simulink model "F16ASYM_Controlled_AoA"  (R2012b)
settings: Solver=ode3  SolverMode=SingleTasking  StartTime=0.0  StopTime=inf  FixedStep=T_sim  RelTol=1e-3
InitFcn:
  | load('NN_c_weights_Last_stable.mat')
values from neighbouring files (symbols this model uses):
  K_b_AoA = params(3)    [Cost_function.m]
  K_b_q = params(4)    [Cost_function.m]
  learning = 20    [Scheduling_desing.m]
  Model_used_flag = 1    [Scheduling_desing.m]
  reg_param = 0.5    [Scheduling_desing.m]
  T_sim = 0.02    [Scheduling_desing.m]
  tau_AoA = params(1)    [Cost_function.m]
  tau_q = params(2)    [Cost_function.m]
  Theta_1_roll_last = [0.00183613313267 0.00115998993235 0.0006676025148 0.00194921904952 0.00134963559861 0.00034352059664 0.000447169388141 0.00146749660935 0.00110199952389 7.77922383894e-05 0.00109492833348 0.00192687590535 ... (360 elements, 30x12)]    [NN_i_weights_LAST_STABLE.mat]
  Theta_2_roll_last = [0.000469743069697 0.000355923851088 0.00180035760697 0.00191855117771 0.00118851504447 0.0013331642065 0.0013164316578 0.000643981263341 0.00176817665434 0.000113802099363 0.000426534542462 0.00113815782354 ... (620 elements, 20x31)]    [NN_i_weights_LAST_STABLE.mat]
  Theta_3_roll_last = [9.62071520568e-05 -0.000389870886846 2.08260845013e-05 0.000140787743673 -0.000917525755397 -0.0014324207578 -0.00154701573815 -0.00131544476264 -0.00101205584381 5.06515794689e-05 -0.00111443483676 -0.00143957416141 ... (21 elements, 1x21)]    [NN_i_weights_LAST_STABLE.mat]
  V_long_lastA_w_z = [0.352826086601 -0.253633004548 -0.642535042878 0.237749930435 -0.618390629538 0.858074761295 0.268211230628 -0.448715080196 -0.0406384631192 0.401147605577 0.60598427709 0.0500551915851 ... (300 elements, 30x10)]    [NN_i_weights_LAST_STABLE.mat]
  V_long_lastAoA = [0.0774300162379 0.0911421319631 0.0352371192557 0.0542170286952 0.0651171200844 0.0177112012707 0.0982957728448 0.000259994642558 0.0194724569123 0.0466321328252 0.0556687953852 0.0252668067142 ... (300 elements, 30x10)]    [NN_i_weights_LAST_STABLE.mat]
  V_roll_last = [0.0540918675943 0.0557493347212 0.0839792276608 0.0460576391794 0.0671229058124 0.100220403067 0.0722493281881 0.0648875457457 0.00447599349201 0.0607299103823 0.0488037966361 0.0176785979393 ... (360 elements, 30x12)]    [NN_i_weights_LAST_STABLE.mat]
  V_yaw_last = [0.0965149149679 0.00833616709545 0.0365734360076 0.0523944217566 0.00790252078455 0.0700053845887 0.0345164868709 0.0111568465295 0.094060639546 0.0205483560006 0.000798047494256 0.0862769385758 ... (360 elements, 30x12)]    [NN_i_weights_LAST_STABLE.mat]
  velocity = M_eval_sche(I,J)*a    [Scheduling_desing.m]
  W_long_lastA_w_z = [-0.0522913429974 0.00385484301394 -0.00465489482472 -0.0139416219936 0.00295196421483 -0.013027768541 0.00585545058915 0.00278802233571 -0.00906272782329 -0.000396112031465 0.00405849743321 0.00509668457818 ... (31 elements, 1x31)]    [NN_i_weights_LAST_STABLE.mat]
  W_long_lastAoA = [-0.0192589013922 0.00873109909713 0.00432649597332 0.0420946902441 0.0293366820194 0.0351497798191 0.0234952374236 0.0360841187718 0.0112233388211 0.030147202199 0.0369533138617 0.00218839076415 ... (31 elements, 1x31)]    [NN_i_weights_LAST_STABLE.mat]
  W_roll_last = [-0.0006515532842 0.000535485585715 0.000550946920743 0.000806030945453 0.00045976209382 0.00065557954304 0.000945902185602 0.00070191398535 0.000635215543728 4.66501377412e-05 0.000597079583757 0.000485790566765 ... (31 elements, 1x31)]    [NN_i_weights_LAST_STABLE.mat]
  W_yaw_last = [-4.34263633305e-05 8.83823048922e-05 1.65575463724e-05 3.60293102233e-05 5.19752447623e-05 7.06399280852e-06 7.02425975821e-05 3.62680255076e-05 1.29996379937e-05 8.05072914397e-05 2.39941870661e-05 2.52427840574e-06 ... (31 elements, 1x31)]    [NN_i_weights_LAST_STABLE.mat]
undefined symbols (not defined in the file or in its folder): a1, alpha_map_eval, B, beta_map_eval, C_L_0, DiscIntNeverNeededParam, fi_flag_Simulink, G_eval, H_sq, H_sq_autotrim, k_B, m_B, M_sq, M_sq_autotrim, sigbuilder_block, Stall_curve, trim_control, trim_state, trim_throttle, V_Comp_A_w_z_last, V_Comp_last, V_roll_lastMOD, W_Comp_A_w_z_last, W_Comp_last, W_roll_lastMOD
libraries: Adaptive_FaultTolerantControl x43, dspsigops x29, F16_Actuator_Library x14, simulink x8, aerolibatmos2 x7, dsparch4 x6, simulink_extras x5, aerolibtransform2 x5, qcatlib x4, dspmtrx3 x3, dspvision x2, dspsnks4 x2
(part 5 of 11)

== system F16ASYM_Controlled_AoA/F-16 Non-linear Plant/SYM and ASYM model: No reconfigurable/Actuators Dynamcis ==
  note: Controls:
      | 1. Throttle
      | 2. Elevator_L in deg
      | 3. Elevator_R in deg
      | 4. Aileron_L
      | 5. Aileron_R
      | 6. Rudder
      | 7. LEF_L
      | 8. LEF_R
  note: Units: deg.
  note: Units: deg.
  note: Units: deg.
  note: This addition in LEFs can be done
      |  if assumed Linear aerodynamics
  note: No dynamics for throttle since the engine dynamics is inside the model
  Control_commands : Inport
  Aileron Actuator : F16_Actuator_Library/Aileron Actuator
  Aileron Actuator1 : F16_Actuator_Library/Aileron Actuator
  Aileron_L Trim Setting : Constant  Value=trim_control(2)
  Aileron_R Trim Setting : Constant  Value=-trim_control(2)
  Control Surface Deflections : ToWorkspace  VariableName=surfaces  SampleTime=-1
      settings: Decimation=100
  Demux : Demux  Outputs=8
  Elevator Actuator : F16_Actuator_Library/Elevator Actuator
  Elevator Actuator1 : F16_Actuator_Library/Elevator Actuator
  LEF Actuator : F16_Actuator_Library/LEF Actuator
  LEF Actuator1 : F16_Actuator_Library/LEF Actuator
  Mux{,1,3..7} (7 alike) : Mux  Inputs=2
  Mux2 : Mux  Inputs=8
  Mux8 : Mux  Inputs=7
  Rudder Actuator : F16_Actuator_Library/Rudder Actuator
  Saturation1 : Saturate  UpperLimit=1  LowerLimit=0
  Control Defl Plot : Outport
  Dec_Control_def : Outport  Port=2
  Throttle_meas : Outport  Port=3
  wires:
  Saturation1/1 -> Mux2/1, Throttle_meas/1  "Throttle"
  Aileron_R Trim Setting/1 -> Aileron Actuator1/2
  Aileron_L Trim Setting/1 -> Aileron Actuator/2
  Demux/1 -> Saturation1/1
  Mux7/1 -> [LEF_R]
  LEF Actuator1/1 -> Mux7/2, Mux2/8  "LEF_R"
  Demux/8 -> Mux7/1, LEF Actuator1/1
  Mux6/1 -> [LEF_L]
  LEF Actuator/1 -> Mux2/7, Mux6/2  "LEF_L"
  Demux/7 -> Mux6/1, LEF Actuator/1
  Mux5/1 -> [Ail_R]
  Aileron Actuator1/1 -> Mux2/5, Mux5/1  "Aileron_R"
  Demux/5 -> Aileron Actuator1/1, Mux5/2
  Elevator Actuator1/1 -> Mux2/3, Mux4/1  "Elevator_R"
  Demux/3 -> Mux4/2, Elevator Actuator1/1
  Mux3/1 -> [Rudder]
  Mux1/1 -> [Ail_L]
  Rudder Actuator/1 -> Mux2/6, Mux3/2  "Rudder"
  Aileron Actuator/1 -> Mux2/4, Mux1/2  "Aileron_L"
  Demux/6 -> Mux3/1, Rudder Actuator/1
  Demux/4 -> Aileron Actuator/1, Mux1/1
  Mux/1 -> [Elev_L]
  Elevator Actuator/1 -> Mux2/2, Mux/2  "Elevator_L"
  Mux2/1 -> Control Surface Deflections/1, Dec_Control_def/1
  Demux/2 -> Elevator Actuator/1, Mux/1
  Control_commands/1 -> Demux/1
  Mux8/1 -> Control Defl Plot/1
  [Elev_L] -> Mux8/1
  [Elev_R] -> Mux8/2
  [Ail_L] -> Mux8/3
  [Ail_R] -> Mux8/4
  [Rudder] -> Mux8/5
  [LEF_L] -> Mux8/6
  [LEF_R] -> Mux8/7
  Mux4/1 -> [Elev_R]

== system F16ASYM_Controlled_AoA/F-16 Non-linear Plant/SYM and ASYM model: No reconfigurable/Leading Edge Flap:Symetric deflection ==
  note: Initialize LF_state with -alpha0 value in degrees!!!!
  note: Same as atmos() in nlplant...c
  note: see NASA Technical Paper 1538, p34
  state : Inport
  Bus Selector1 : BusSelector  OutputSignals=X_e,TAS,alpha;beta
  Creating    qbar / ps : Subsystem
  Demux1 : Demux  Outputs=2
  Gain : Gain  Gain=2  SaturateOnIntegerOverflow=on  OutDataTypeStr=Inherit: Same as input  ParamDataTypeStr=Inherit: Same as input
  Gain1 : Gain  Gain=7.25  SaturateOnIntegerOverflow=on  OutDataTypeStr=Inherit: Same as input  ParamDataTypeStr=Inherit: Same as input
  Gain2 : Gain  Gain=1.38  SaturateOnIntegerOverflow=on  OutDataTypeStr=Inherit: Same as input  ParamDataTypeStr=Inherit: Same as input
  LF_state : Integrator  InitialCondition=-trim_state(8)*180/pi
  Selector : Selector  InputPortWidth=3  IndexOptions=Index vector (dialog)  Indices=3  OutputSizes=1
  Sum : Sum  Inputs=-|+|+  SaturateOnIntegerOverflow=on  InputSameDT=on  OutDataTypeStr=Inherit: Same as first input
  Sum1 : Sum  Inputs=|+-  SaturateOnIntegerOverflow=on  InputSameDT=on  OutDataTypeStr=Inherit: Same as first input
  Sum2 : Sum  Inputs=++|  SaturateOnIntegerOverflow=on  InputSameDT=on  OutDataTypeStr=Inherit: Same as first input
  coeff1 : Constant  Value=1.45
  r2d1 : Gain  Gain=180/pi  SaturateOnIntegerOverflow=on  OutDataTypeStr=Inherit: Same as input  ParamDataTypeStr=Inherit: Same as input
  r2d6 : Gain  Gain=9.05  SaturateOnIntegerOverflow=on  OutDataTypeStr=Inherit: Same as input  ParamDataTypeStr=Inherit: Same as input
  delta_lef (deg) : Outport
  wires:
  Bus Selector1/3 -> Demux1/1  "<alpha;beta>"
  Bus Selector1/1 -> Selector/1  "<X_e>"
  r2d6/1 -> Sum/1
  Creating    qbar / ps/1(qbar / ps) -> r2d6/1
  Bus Selector1/2 -> Creating    qbar / ps/2(V)  "<TAS>"
  r2d1/1 -> Gain/1, Sum1/1  "alpha"
  LF_state/1 -> Sum2/2
  Sum2/1 -> Gain2/1, Sum1/2
  coeff1/1 -> Sum/3
  Demux1/1 -> r2d1/1
  Gain2/1 -> Sum/2
  Gain/1 -> Sum2/1
  Gain1/1 -> LF_state/1
  Sum1/1 -> Gain1/1
  state/1 -> Bus Selector1/1
  Sum/1 -> delta_lef (deg)/1
  Selector/1 -> Creating    qbar / ps/1(alt)

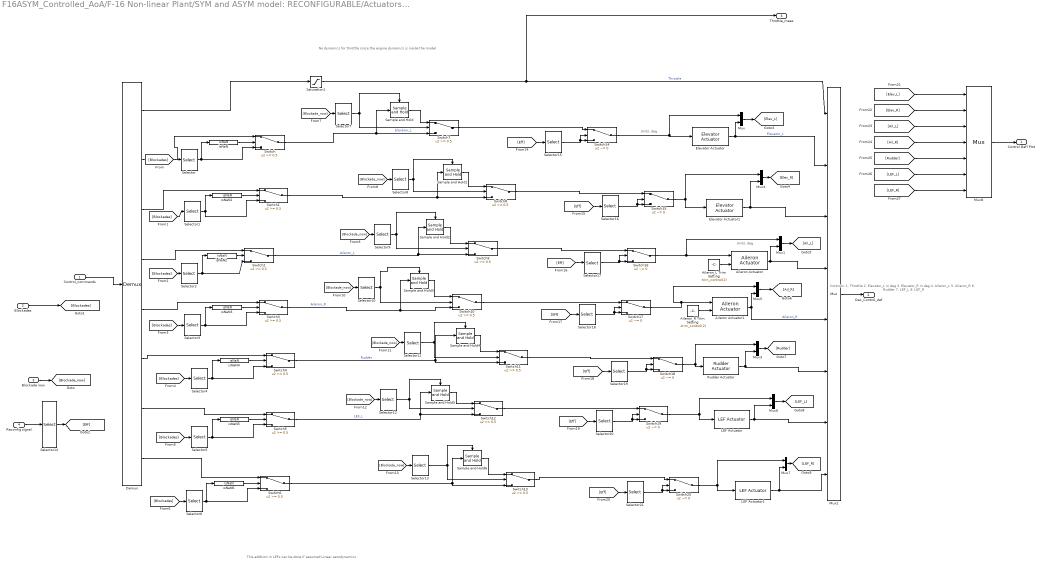
== system F16ASYM_Controlled_AoA/F-16 Non-linear Plant/SYM and ASYM model: RECONFIGURABLE/Actuators Dynamcis ==
  note: No dynamics for throttle since the engine dynamics is inside the model
  note: This addition in LEFs can be done
      |  if assumed Linear aerodynamics
  note: Units: deg.
  note: Units: deg.
  note: Controls:
      | 1. Throttle
      | 2. Elevator_L in deg
      | 3. Elevator_R in deg
      | 4. Aileron_L
      | 5. Aileron_R
      | 6. Rudder
      | 7. LEF_L
      | 8. LEF_R
  Control_commands : Inport
  Blockades : Inport  Port=2
  Blockade now : Inport  Port=3
  Reconfig signal : Inport  Port=4
  Aileron Actuator : F16_Actuator_Library/Aileron Actuator
  Aileron Actuator1 : F16_Actuator_Library/Aileron Actuator
  Aileron_L Trim Setting : Constant  Value=trim_control(2)
  Aileron_R Trim Setting : Constant  Value=-trim_control(2)
  Demux : Demux  Outputs=8
  Elevator Actuator : F16_Actuator_Library/Elevator Actuator
  Elevator Actuator1 : F16_Actuator_Library/Elevator Actuator
  LEF Actuator : F16_Actuator_Library/LEF Actuator
  LEF Actuator1 : F16_Actuator_Library/LEF Actuator
  Mux{,1,3..7} (7 alike) : Mux  Inputs=2
  Mux2 : Mux  Inputs=8
  Mux8 : Mux  Inputs=7
  Rudder Actuator : F16_Actuator_Library/Rudder Actuator
  Sample and Hold : dspsigops/Sample and Hold  trig=Rising edge  initCond=trim_control(1)  latchinput=off
  Sample and Hold1 : dspsigops/Sample and Hold  trig=Rising edge  initCond=trim_control(1)  latchinput=off
  Sample and Hold2 : dspsigops/Sample and Hold  trig=Rising edge  initCond=trim_control(2)  latchinput=off
  Sample and Hold3 : dspsigops/Sample and Hold  trig=Rising edge  initCond=-trim_control(2)  latchinput=off
  Sample and Hold4 : dspsigops/Sample and Hold  trig=Rising edge  initCond=trim_control(3)  latchinput=off
  Sample and Hold5 : dspsigops/Sample and Hold  trig=Rising edge  initCond=dLEF  latchinput=off
  Sample and Hold6 : dspsigops/Sample and Hold  trig=Rising edge  initCond=dLEF  latchinput=off
  Saturation1 : Saturate  UpperLimit=1  LowerLimit=0
  Selector : Selector  InputPortWidth=7  IndexOptions=Index vector (dialog)  Indices=1  OutputSizes=1
  Selector1 : Selector  InputPortWidth=7  IndexOptions=Index vector (dialog)  Indices=2  OutputSizes=1
  Selector10 : Selector  InputPortWidth=7  IndexOptions=Index vector (dialog)  Indices=4  OutputSizes=1
  Selector11 : Selector  InputPortWidth=7  IndexOptions=Index vector (dialog)  Indices=5  OutputSizes=1
  Selector12 : Selector  InputPortWidth=7  IndexOptions=Index vector (dialog)  Indices=6  OutputSizes=1
  Selector13 : Selector  InputPortWidth=7  IndexOptions=Index vector (dialog)  Indices=7  OutputSizes=1
  Selector14 : Selector  InputPortWidth=19  IndexOptions=Index vector (dialog)  Indices=10:16  OutputSizes=1
  Selector15 : Selector  InputPortWidth=7  IndexOptions=Index vector (dialog)  Indices=1  OutputSizes=1
  Selector16 : Selector  InputPortWidth=7  IndexOptions=Index vector (dialog)  Indices=2  OutputSizes=1
  Selector17 : Selector  InputPortWidth=7  IndexOptions=Index vector (dialog)  Indices=3  OutputSizes=1
  Selector18 : Selector  InputPortWidth=7  IndexOptions=Index vector (dialog)  Indices=4  OutputSizes=1
  Selector19 : Selector  InputPortWidth=7  IndexOptions=Index vector (dialog)  Indices=5  OutputSizes=1
  Selector2 : Selector  InputPortWidth=7  IndexOptions=Index vector (dialog)  Indices=3  OutputSizes=1
  Selector20 : Selector  InputPortWidth=7  IndexOptions=Index vector (dialog)  Indices=6  OutputSizes=1
  Selector21 : Selector  InputPortWidth=7  IndexOptions=Index vector (dialog)  Indices=7  OutputSizes=1
  Selector3 : Selector  InputPortWidth=7  IndexOptions=Index vector (dialog)  Indices=4  OutputSizes=1
  Selector4 : Selector  InputPortWidth=7  IndexOptions=Index vector (dialog)  Indices=5  OutputSizes=1
  Selector5 : Selector  InputPortWidth=7  IndexOptions=Index vector (dialog)  Indices=6  OutputSizes=1
  Selector6 : Selector  InputPortWidth=7  IndexOptions=Index vector (dialog)  Indices=7  OutputSizes=1
  Selector7 : Selector  InputPortWidth=7  IndexOptions=Index vector (dialog)  Indices=1  OutputSizes=1
  Selector8 : Selector  InputPortWidth=7  IndexOptions=Index vector (dialog)  Indices=2  OutputSizes=1
  Selector9 : Selector  InputPortWidth=7  IndexOptions=Index vector (dialog)  Indices=3  OutputSizes=1
  Switch{,1..13} (14 alike) : Switch  Threshold=0.5
  Switch{14..20} (7 alike) : Switch  Criteria=u2 ~= 0
  isNaN{,1..6} (7 alike) : RelationalOperator  Operator=isNaN  OutDataTypeStr=boolean
  Control Defl Plot : Outport
  Dec_Control_def : Outport  Port=2
  Throttle_meas : Outport  Port=3
  wires:
  Control_commands/1 -> Demux/1
  Switch14/1 -> Elevator Actuator/1, Mux/1
  Mux2/1 -> Dec_Control_def/1
  Switch16/1 -> Mux1/1, Aileron Actuator/1
  Switch18/1 -> Mux3/1, Rudder Actuator/1
  Switch19/1 -> Mux6/1, LEF Actuator/1
  Switch20/1 -> Mux7/1, LEF Actuator1/1
  Demux/1 -> Saturation1/1
  Aileron_L Trim Setting/1 -> Aileron Actuator/2
  Aileron_R Trim Setting/1 -> Aileron Actuator1/2
  Saturation1/1 -> Mux2/1, Throttle_meas/1  "Throttle"
  Blockades/1 -> [Blockades]
  Blockade now/1 -> [Blockade_now]
  [Blockades] -> Selector/1
  isNaN/1 -> Switch/2
  Demux/2 -> Switch/1
  Selector/1 -> Switch/3, isNaN/1
  [Blockades] -> Selector1/1
  isNaN1/1 -> Switch1/2
  Demux/3 -> Switch1/1
  Selector1/1 -> Switch1/3, isNaN1/1
  [Blockades] -> Selector2/1
  isNaN2/1 -> Switch2/2
  Demux/4 -> Switch2/1
  Selector2/1 -> Switch2/3, isNaN2/1
  [Blockades] -> Selector3/1
  isNaN3/1 -> Switch3/2
  Demux/5 -> Switch3/1
  Selector3/1 -> Switch3/3, isNaN3/1
  [Blockades] -> Selector4/1
  isNaN4/1 -> Switch4/2
  Demux/6 -> Switch4/1
  Selector4/1 -> Switch4/3, isNaN4/1
  [Blockades] -> Selector5/1
  isNaN5/1 -> Switch5/2
  Demux/7 -> Switch5/1
  Selector5/1 -> Switch5/3, isNaN5/1
  [Blockades] -> Selector6/1
  isNaN6/1 -> Switch6/2
  Demux/8 -> Switch6/1
  Selector6/1 -> Switch6/3, isNaN6/1
  Aileron Actuator/1 -> Mux2/4, Mux1/2
  Rudder Actuator/1 -> Mux3/2, Mux2/6
  LEF Actuator/1 -> Mux2/7, Mux6/2
  Switch/1 -> Switch7/3, Sample and Hold/1  "Elevator_L"
  [Blockade_now] -> Selector7/1
  Sample and Hold/1 -> Switch7/1
  Selector7/1 -> Switch7/2, Sample and Hold/Trigger
  Elevator Actuator/1 -> Mux/2, Mux2/2  "Elevator_L"
  Switch1/1 -> Sample and Hold1/1, Switch8/3
  [Blockade_now] -> Selector8/1
  Sample and Hold1/1 -> Switch8/1
  Selector8/1 -> Switch8/2, Sample and Hold1/Trigger
  Switch15/1 -> Mux4/1, Elevator Actuator1/1
  Switch2/1 -> Sample and Hold2/1, Switch9/3  "Aileron_L"
  [Blockade_now] -> Selector9/1
  Sample and Hold2/1 -> Switch9/1
  Selector9/1 -> Sample and Hold2/Trigger, Switch9/2
  Switch17/1 -> Mux5/1, Aileron Actuator1/1
  Aileron Actuator1/1 -> Mux2/5, Mux5/2  "Aileron_R"
  Switch3/1 -> Switch10/3, Sample and Hold3/1  "Aileron_R"
  [Blockade_now] -> Selector10/1
  Sample and Hold3/1 -> Switch10/1
  Selector10/1 -> Sample and Hold3/Trigger, Switch10/2
  Switch4/1 -> Switch11/3, Sample and Hold4/1  "Rudder"
  [Blockade_now] -> Selector11/1
  Sample and Hold4/1 -> Switch11/1
  Selector11/1 -> Switch11/2, Sample and Hold4/Trigger
  Switch5/1 -> Sample and Hold5/1, Switch12/3  "LEF_L"
  [Blockade_now] -> Selector12/1
  Sample and Hold5/1 -> Switch12/1
  Selector12/1 -> Switch12/2, Sample and Hold5/Trigger
  LEF Actuator1/1 -> Mux7/2, Mux2/8
  Switch6/1 -> Switch13/3, Sample and Hold6/1
  [Blockade_now] -> Selector13/1
  Sample and Hold6/1 -> Switch13/1
  Selector13/1 -> Switch13/2, Sample and Hold6/Trigger
  Elevator Actuator1/1 -> Mux4/2, Mux2/3
  Reconfig signal/1 -> Selector14/1
  Selector14/1 -> [Eff]
  [Eff] -> Selector15/1
  Switch7/1 -> Switch14/1
  Selector15/1 -> Switch14/2, Switch14/3
  [Eff] -> Selector16/1
  Switch8/1 -> Switch15/1
  Selector16/1 -> Switch15/2, Switch15/3
  [Eff] -> Selector17/1
  Switch9/1 -> Switch16/1
  Selector17/1 -> Switch16/2, Switch16/3
  [Eff] -> Selector18/1
  Switch10/1 -> Switch17/1
  Selector18/1 -> Switch17/2, Switch17/3
  [Eff] -> Selector19/1
  Switch11/1 -> Switch18/1
  Selector19/1 -> Switch18/2, Switch18/3
  [Eff] -> Selector20/1
  Switch12/1 -> Switch19/1
  Selector20/1 -> Switch19/2, Switch19/3
  [Eff] -> Selector21/1
  Switch13/1 -> Switch20/1
  Selector21/1 -> Switch20/2, Switch20/3
  Mux/1 -> [Elev_L]
  Mux4/1 -> [Elev_R]
  Mux1/1 -> [Ail_L]
  Mux5/1 -> [Ail_R]
  Mux3/1 -> [Rudder]
  Mux6/1 -> [LEF_L]
  Mux7/1 -> [LEF_R]
  Mux8/1 -> Control Defl Plot/1
  [Elev_L] -> Mux8/1
  [Elev_R] -> Mux8/2
  [Ail_L] -> Mux8/3
  [Ail_R] -> Mux8/4
  [Rudder] -> Mux8/5
  [LEF_L] -> Mux8/6
  [LEF_R] -> Mux8/7

== system F16ASYM_Controlled_AoA/F-16 Non-linear Plant/SYM and ASYM model: RECONFIGURABLE/Leading Edge Flap:Symetric deflection ==
  note: see NASA Technical Paper 1538, p34
  note: Same as atmos() in nlplant...c
  note: Initialize LF_state with -alpha0 value in degrees!!!!
  state : Inport
  Bus Selector1 : BusSelector  OutputSignals=X_e,TAS,alpha ; beta
  Creating    qbar / ps : Subsystem
  Gain : Gain  Gain=2  SaturateOnIntegerOverflow=on  OutDataTypeStr=Inherit: Same as input  ParamDataTypeStr=Inherit: Same as input
  Gain1 : Gain  Gain=7.25  SaturateOnIntegerOverflow=on  OutDataTypeStr=Inherit: Same as input  ParamDataTypeStr=Inherit: Same as input
  Gain2 : Gain  Gain=1.38  SaturateOnIntegerOverflow=on  OutDataTypeStr=Inherit: Same as input  ParamDataTypeStr=Inherit: Same as input
  LF_state : Integrator  InitialCondition=-trim_state(8)*180/pi
  Selector : Selector  InputPortWidth=3  IndexOptions=Index vector (dialog)  Indices=3  OutputSizes=1
  Selector1 : Selector  InputPortWidth=2  IndexOptions=Index vector (dialog)  Indices=1  OutputSizes=1
  Sum : Sum  Inputs=-|+|+  SaturateOnIntegerOverflow=on  InputSameDT=on  OutDataTypeStr=Inherit: Same as first input
  Sum1 : Sum  Inputs=|+-  SaturateOnIntegerOverflow=on  InputSameDT=on  OutDataTypeStr=Inherit: Same as first input
  Sum2 : Sum  Inputs=++|  SaturateOnIntegerOverflow=on  InputSameDT=on  OutDataTypeStr=Inherit: Same as first input
  coeff1 : Constant  Value=1.45
  r2d1 : Gain  Gain=180/pi  SaturateOnIntegerOverflow=on  OutDataTypeStr=Inherit: Same as input  ParamDataTypeStr=Inherit: Same as input
  r2d6 : Gain  Gain=9.05  SaturateOnIntegerOverflow=on  OutDataTypeStr=Inherit: Same as input  ParamDataTypeStr=Inherit: Same as input
  delta_lef (deg) : Outport
  wires:
  Sum/1 -> delta_lef (deg)/1
  state/1 -> Bus Selector1/1
  Sum1/1 -> Gain1/1
  Gain1/1 -> LF_state/1
  Gain/1 -> Sum2/1
  Gain2/1 -> Sum/2
  Selector1/1 -> r2d1/1
  coeff1/1 -> Sum/3
  Sum2/1 -> Sum1/2, Gain2/1
  LF_state/1 -> Sum2/2
  r2d1/1 -> Sum1/1, Gain/1  "alpha"
  Bus Selector1/2 -> Creating    qbar / ps/2(V)  "<TAS>"
  Creating    qbar / ps/1(qbar / ps) -> r2d6/1
  r2d6/1 -> Sum/1
  Bus Selector1/3 -> Selector1/1  "<alpha ; beta>"
  Bus Selector1/1 -> Selector/1  "<X_e>"
  Selector/1 -> Creating    qbar / ps/1(alt)

== system F16ASYM_Controlled_AoA/NDI/NDI: NO RECONFIG/Dim_less ==
  L_comm : Inport
  M_comm : Inport  Port=2
  N_comm : Inport  Port=3
  q : Inport  Port=4
  B span : Constant  Value=9.144
  CMA : Constant  Value=3.45
  Divide : Product  Inputs=*/
  Divide1 : Product  Inputs=***
  Divide2 : Product  Inputs=/*
  Divide3 : Product  Inputs=***
  Divide4 : Product  Inputs=*/
  S_w : Constant  Value=27.87
  S_w1 : Constant  Value=27.87
  q1 : InportShadow  Port=4
  C_L des : Outport
  C_M des : Outport  Port=2
  C_N des : Outport  Port=3
  wires:
  Divide4/1 -> C_M des/1  "C_M"
  Divide3/1 -> Divide4/2
  M_comm/1 -> Divide4/1
  CMA/1 -> Divide3/3
  S_w1/1 -> Divide3/2
  q1/1 -> Divide3/1
  Divide2/1 -> C_N des/1  "C_N"
  N_comm/1 -> Divide2/2
  Divide/1 -> C_L des/1  "C_L"
  Divide1/1 -> Divide/2, Divide2/1
  L_comm/1 -> Divide/1
  B span/1 -> Divide1/3
  S_w/1 -> Divide1/2
  q/1 -> Divide1/1

== system F16ASYM_Controlled_AoA/NDI/NDI: RECONFIG/Dim_less ==
  L_comm : Inport
  M_comm : Inport  Port=2
  N_comm : Inport  Port=3
  q : Inport  Port=4
  B span : Constant  Value=9.144
  CMA : Constant  Value=3.45
  Divide : Product  Inputs=*/
  Divide1 : Product  Inputs=***
  Divide2 : Product  Inputs=/*
  Divide3 : Product  Inputs=***
  Divide4 : Product  Inputs=*/
  S_w : Constant  Value=27.87
  S_w1 : Constant  Value=27.87
  q1 : InportShadow  Port=4
  C_L des : Outport
  C_M des : Outport  Port=2
  C_N des : Outport  Port=3
  wires:
  q/1 -> Divide1/1
  S_w/1 -> Divide1/2
  B span/1 -> Divide1/3
  L_comm/1 -> Divide/1
  Divide1/1 -> Divide2/1, Divide/2
  Divide/1 -> C_L des/1  "C_L"
  N_comm/1 -> Divide2/2
  Divide2/1 -> C_N des/1  "C_N"
  q1/1 -> Divide3/1
  S_w1/1 -> Divide3/2
  CMA/1 -> Divide3/3
  M_comm/1 -> Divide4/1
  Divide3/1 -> Divide4/2
  Divide4/1 -> C_M des/1  "C_M"

== system F16ASYM_Controlled_AoA/P controller + adaptive Crossed NN + AWU+Lim+scheduling   in AoA/Body Rates Controller/Ref Model and P Controller q ==
  y_ref : Inport
  y_meas : Inport  Port=2
  " " : Sum  Inputs=|+-
  Add1 : Sum  Inputs=++|
  Divide : Product  Inputs=**
  K_b params : Constant  Value=K_b_q
  K_f : Gain
  Reference Model : Subsystem
  y_des_dot : Outport
  y_c_ff_dot : Outport  Port=2
  y_c : Outport  Port=3
  y_meas_out : Outport  Port=4
  k_b param : Outport  Port=5
  wires:
  K_b params/1 -> k_b param/1, Divide/2
  y_meas/1 -> y_meas_out/1, " "/2
  Reference Model/2(y_c) -> y_c/1, " "/1
  " "/1 -> Divide/1
  y_ref/1 -> Reference Model/1(y_ref)
  Add1/1 -> y_des_dot/1
  Reference Model/1(y_c_dot) -> K_f/1
  K_f/1 -> y_c_ff_dot/1, Add1/1
  Divide/1 -> Add1/2

== system F16ASYM_Controlled_AoA/P controller + adaptive Crossed NN + AWU+Lim+scheduling   in AoA/Long Dyn Inversion: alpha_dot ->q/Completed ==
  alpha_dot_c : Inport
  All_meas : Inport  Port=2
  A_w_z : Selector  InputPortWidth=3  IndexOptions=Index vector (dialog)  Indices=3  OutputSizes=1
  Add : Sum
  Bus Selector : BusSelector  OutputSignals=signal1.AoA meas (rad),signal1.omega_b meas (rad/s),signal1.SS meas (rad),signal1.V_TAS (m/s),signal2.A_w_CG
  Display : Display
  Display1 : Display
  Display2 : Display
  Divide{,1..3} (4 alike) : Product  Inputs=**
  Divide4 : Product  Inputs=/*
  Selector : Selector  InputPortWidth=3  IndexOptions=Index vector (dialog)  Indices=1  OutputSizes=1
  Selector1 : Selector  InputPortWidth=3  IndexOptions=Index vector (dialog)  Indices=3  OutputSizes=1
  Trigonometric Function : Trigonometry  Operator=sincos
  Trigonometric Function1 : Trigonometry  Operator=tan
  Trigonometric Function2 : Trigonometry  Operator=cos
  "q_c " : Sum  Inputs=++-
  q_c : Outport
  wires:
  Trigonometric Function/1 -> Divide1/1
  Bus Selector/1 -> Trigonometric Function/1  "<AoA meas (rad)>"
  Selector/1 -> Divide/2
  Bus Selector/2 -> Selector1/1, Selector/1  "<omega_b meas (rad/s)>"
  Divide2/1 -> "q_c "/2, Display1/1
  Selector1/1 -> Divide1/2
  Divide3/1 -> Divide4/1
  alpha_dot_c/1 -> "q_c "/1, Display/1
  All_meas/1 -> Bus Selector/1
  Bus Selector/5 -> A_w_z/1  "<A_w_CG>"
  Bus Selector/3 -> Trigonometric Function1/1, Trigonometric Function2/1  "<SS meas (rad)>"
  Divide4/1 -> "q_c "/3
  "q_c "/1 -> q_c/1
  Divide/1 -> Add/1
  Bus Selector/4 -> Divide3/2  "<V_TAS (m/s)>"
  Add/1 -> Divide2/1
  Trigonometric Function1/1 -> Divide2/2
  Divide1/1 -> Add/2
  Trigonometric Function2/1 -> Divide3/1
  Trigonometric Function/2 -> Divide/1
  A_w_z/1 -> Display2/1, Divide4/2

== system F16ASYM_Controlled_AoA/P controller + adaptive Crossed NN + AWU+Lim+scheduling   in AoA/Long Dyn Inversion: alpha_dot ->q/Simplified ==
  alpha_dot_c : Inport
  All_meas : Inport  Port=2
  A_b_z : Selector  InputPortWidth=3  IndexOptions=Index vector (dialog)  Indices=3  OutputSizes=1
  Bus Selector : BusSelector  OutputSignals=signal2.A_b_CG,signal1.V_TAS (m/s)
  Display : Display
  Divide4 : Product  Inputs=*/
  "q_c " : Sum  Inputs=+-
  q_c : Outport
  wires:
  "q_c "/1 -> q_c/1
  All_meas/1 -> Bus Selector/1
  alpha_dot_c/1 -> "q_c "/1, Display/1
  Bus Selector/2 -> Divide4/2  "<V_TAS (m/s)>"
  Divide4/1 -> "q_c "/2
  A_b_z/1 -> Divide4/1  "A_b_z"
  Bus Selector/1 -> A_b_z/1  "<A_b_CG>"

== system F16ASYM_Controlled_AoA/P controller + adaptive Crossed NN + AWU+Lim+scheduling   in AoA/Longitudinal controller in AoA/Ref Model and P Controller ==
  y_ref : Inport
  y_meas : Inport  Port=2
  " " : Sum  Inputs=|+-
  Add1 : Sum  Inputs=++|
  Divide : Product  Inputs=**
  K_b params : Constant  Value=K_b_AoA
  K_f : Gain
  Reference Model : Subsystem
  y_des_dot : Outport
  y_c_ff_dot : Outport  Port=2
  y_c : Outport  Port=3
  y_meas_out : Outport  Port=4
  k_b param : Outport  Port=5
  wires:
  K_b params/1 -> k_b param/1, Divide/2
  y_meas/1 -> y_meas_out/1, " "/2
  Reference Model/2(y_c) -> y_c/1, " "/1
  " "/1 -> Divide/1
  y_ref/1 -> Reference Model/1(y_ref)
  Add1/1 -> y_des_dot/1
  Reference Model/1(y_c_dot) -> K_f/1
  K_f/1 -> y_c_ff_dot/1, Add1/1
  Divide/1 -> Add1/2

== system F16ASYM_Controlled_AoA/P controller + adaptive Crossed NN + AWU+Lim+scheduling   in AoA/Physical limitation/Moments ==
  C_L : Inport
  C_M : Inport  Port=2
  C_N : Inport  Port=3
  q : Inport  Port=4
  B span : Constant  Value=9.144
  CMA : Constant  Value=3.45
  Divide : Product  Inputs=**
  Divide1 : Product  Inputs=***
  Divide2 : Product  Inputs=**
  Divide3 : Product  Inputs=***
  Divide4 : Product  Inputs=**
  S_w : Constant  Value=27.87
  S_w1 : Constant  Value=27.87
  q1 : InportShadow  Port=4
  L : Outport
  M : Outport  Port=2
  N : Outport  Port=3
  wires:
  Divide4/1 -> M/1  "M"
  Divide3/1 -> Divide4/2
  C_M/1 -> Divide4/1
  CMA/1 -> Divide3/3
  S_w1/1 -> Divide3/2
  q1/1 -> Divide3/1
  Divide2/1 -> N/1  "N"
  C_N/1 -> Divide2/2
  Divide/1 -> L/1  "L"
  Divide1/1 -> Divide/2, Divide2/1
  C_L/1 -> Divide/1
  B span/1 -> Divide1/3
  S_w/1 -> Divide1/2
  q/1 -> Divide1/1

== system F16ASYM_Controlled_AoA/Primary Controller/P  + Crossed NN + AWU+Lim + hand-over/P controller + adaptive Crossed NN + AWU+Lim    in ACC  ==
  A_w_z des : Inport
  AoA des (rad) : Inport  Port=2
  p des (rad/s) : Inport  Port=3
  beta des (rad) : Inport  Port=4
  Anti-windup A_w_z : Inport  Port=5
  Anti-windup AoA : Inport  Port=6
  Anti-windup beta : Inport  Port=7
  All measures : Inport  Port=8
  Anti-windup signals : Inport  Port=9
  Active : Inport  Port=10
  Body Rates Controller : Subsystem
  Bus Creator : BusCreator  Inputs=3
  Bus Creator1 : BusCreator  Inputs=2
  Bus Creator2 : BusCreator
  Bus Creator3 : BusCreator  Inputs=2
  Bus Selector3 : BusSelector  OutputSignals=signal1.SS meas (rad)
  Complete crossed On-line (adaptive) multi-layer NN: A_w_z : Subsystem  VariantObject=NN on A_w_z
  Display{,1..3,5..6} (6 alike) : Display
  "Display4 " : Display
  Lat_dir Dyn Inversion: beta_dot->r_c : Subsystem
  Long Dyn Inversion: alpha_dot ->q : Subsystem
  Longitudinal controller in A_w_z : Subsystem  VariantObject=Controller of A_w_z
  Memory : Memory  X0=[0,0,0]
  Physical limitation : Subsystem
  Ref Model and P Controller : Adaptive_FaultTolerantControl/Ref Model and P Controller  tau=0.45  y_i=trim_state(9)  K_f=1  K_b=5
  Scope1 : Scope
      settings: TimeRange=10  YMin=-1  YMax=1  SaveName=ScopeData27
  "Sigmoid " : Subsystem  mask{a=0.15}
      mask prompts: a "Sigmoid a param"
      mask TypeOptions a: a/Value
      mask Display:
      | x=-25:0.1:25;
      | 
      | y=(2.0 ./ (1.0 + exp(-a.*x))-1) ;
      | y2=zeros(size(x));
      | 
      | plot(x,y,x,y2);
      | 
      | text(-12,0.5, ['a= ',num2str(a)])
  Sum : Sum  Inputs=-+|
  Sum1 : Sum  Inputs=+-|
  Terminator1 : Terminator
  Angular acc des : Outport
  wires:
  Lat_dir Dyn Inversion: beta_dot->r_c/1(r_c) -> Display6/1, Body Rates Controller/3(r_ref)
  Bus Selector3/1 -> Ref Model and P Controller/2  "<SS meas (rad)>"
  p des (rad/s)/1 -> Body Rates Controller/1(p_ref)
  Long Dyn Inversion: alpha_dot ->q/1(q_c) -> Body Rates Controller/2(q_ref), Display1/1
  beta des (rad)/1 -> Ref Model and P Controller/1
  Longitudinal controller in A_w_z/2(alpha_dot_c) -> Long Dyn Inversion: alpha_dot ->q/1(alpha_dot_c), Display/1
  AoA des (rad)/1 -> Longitudinal controller in A_w_z/2(AoA des (rad))
  Anti-windup AoA/1 -> Longitudinal controller in A_w_z/4(Anti-windup AoA)
  Anti-windup A_w_z/1 -> Longitudinal controller in A_w_z/3(Anti-windup A_w_z)
  A_w_z des/1 -> Longitudinal controller in A_w_z/1(A_w_z des)
  Sum/1 -> "Display4 "/1, "Sigmoid "/1(In), Physical limitation/1(v comm)  "v"
  All measures/1 -> Complete crossed On-line (adaptive) multi-layer NN: A_w_z/2(All_meas), Physical limitation/2(all meas), Body Rates Controller/4(All_meas), Lat_dir Dyn Inversion: beta_dot->r_c/2(All_meas), Bus Selector3/1, Long Dyn Inversion: alpha_dot ->q/2(All_meas), Longitudinal controller in A_w_z/5(All meas)
  Body Rates Controller/4(Angular acc des (rad/s^2)) -> Display3/1, Sum/2  "v_p+v_dot_ff"
  Bus Creator/1 -> Complete crossed On-line (adaptive) multi-layer NN: A_w_z/3(NN variables)
  Memory/1 -> Complete crossed On-line (adaptive) multi-layer NN: A_w_z/1(v_ad^ prev)
  Body Rates Controller/2(p_chanel vars) -> Bus Creator/2  "p_chanel_vars"
  Body Rates Controller/1(q_chanel vars) -> Bus Creator1/2  "q_chanel_vars"
  Longitudinal controller in A_w_z/1(A_chanel vars) -> Bus Creator1/1  "A_chanel vars"
  Bus Creator1/1 -> Bus Creator/1  "Long chanel"
  Ref Model and P Controller/2 -> Bus Creator2/1  "beta_sf_dot"
  Ref Model and P Controller/3 -> Sum1/1, Bus Creator2/2  "beta_sf"
  Sum1/1 -> Bus Creator2/3  "beta_err"
  Ref Model and P Controller/4 -> Sum1/2
  Ref Model and P Controller/5 -> Bus Creator2/4  "K_b_beta"
  Body Rates Controller/3(r_chanel vars) -> Bus Creator3/1  "r_chanel vars"
  Bus Creator2/1 -> Bus Creator3/2  "beta_chanel vars"
  Bus Creator3/1 -> Bus Creator/3  "beta_r_chanel"
  Anti-windup beta/1 -> Terminator1/1
  "Sigmoid "/1(Out) -> Memory/1
  Complete crossed On-line (adaptive) multi-layer NN: A_w_z/1(v_ad^) -> Scope1/1, Display2/1, Sum/1  "v_ad^"
  Ref Model and P Controller/1 -> Display5/1, Lat_dir Dyn Inversion: beta_dot->r_c/1(beta_dot_c)
  Anti-windup signals/1 -> Complete crossed On-line (adaptive) multi-layer NN: A_w_z/4(AWU)
  Physical limitation/1(v limted) -> Angular acc des/1
  Active/1 -> Complete crossed On-line (adaptive) multi-layer NN: A_w_z/Enable

== system F16ASYM_Controlled_AoA/Primary Controller/P  + Crossed NN + AWU+Lim + hand-over/P controller + adaptive Crossed NN + AWU+Lim   in AoA ==
  A_w_z des : Inport
  AoA des (rad) : Inport  Port=2
  p des (rad/s) : Inport  Port=3
  beta des (rad) : Inport  Port=4
  Anti-windup A_w_z : Inport  Port=5
  Anti-windup AoA : Inport  Port=6
  Anti-windup beta : Inport  Port=7
  All measures : Inport  Port=8
  Anti-windup signals : Inport  Port=9
  Active : Inport  Port=10
  Body Rates Controller : Subsystem
  Bus Creator : BusCreator  Inputs=3
  Bus Creator1 : BusCreator  Inputs=2
  Bus Creator2 : BusCreator
  Bus Creator3 : BusCreator  Inputs=2
  Bus Selector3 : BusSelector  OutputSignals=signal1.SS meas (rad)
  Complete crossed On-line (adaptive) multi-layer NN: AoA : Subsystem  VariantObject=NN on AoA
  Display{,1..3,5..6} (6 alike) : Display
  "Display4 " : Display
  Lat_dir Dyn Inversion: beta_dot->r_c : Subsystem
  Long Dyn Inversion: alpha_dot ->q : Subsystem
  Longitudinal controller in AoA : Subsystem  VariantObject=Controller of AoA
  Memory : Memory  X0=[0,0,0]
  Physical limitation : Subsystem
  Ref Model and P Controller : Adaptive_FaultTolerantControl/Ref Model and P Controller  tau=0.45  y_i=trim_state(9)  K_f=1  K_b=5
  Scope1 : Scope
      settings: YMin=-8000  YMax=9000  SaveName=ScopeData27
  "Sigmoid " : Subsystem  mask{a=0.15}
      mask prompts: a "Sigmoid a param"
      mask TypeOptions a: a/Value
      mask Display:
      | x=-25:0.1:25;
      | 
      | y=(2.0 ./ (1.0 + exp(-a.*x))-1) ;
      | y2=zeros(size(x));
      | 
      | plot(x,y,x,y2);
      | 
      | text(-12,0.5, ['a= ',num2str(a)])
  Sum : Sum  Inputs=-+|
  Sum1 : Sum  Inputs=+-|
  Terminator1 : Terminator
  Angular acc des : Outport
  wires:
  Lat_dir Dyn Inversion: beta_dot->r_c/1(r_c) -> Display6/1, Body Rates Controller/3(r_ref)
  Bus Selector3/1 -> Ref Model and P Controller/2  "<SS meas (rad)>"
  p des (rad/s)/1 -> Body Rates Controller/1(p_ref)
  Long Dyn Inversion: alpha_dot ->q/1(q_c) -> Body Rates Controller/2(q_ref), Display1/1
  beta des (rad)/1 -> Ref Model and P Controller/1
  Longitudinal controller in AoA/2(alpha_dot_c) -> Long Dyn Inversion: alpha_dot ->q/1(alpha_dot_c), Display/1
  AoA des (rad)/1 -> Longitudinal controller in AoA/2(AoA des (rad))
  Anti-windup AoA/1 -> Longitudinal controller in AoA/4(Anti-windup AoA)
  Anti-windup A_w_z/1 -> Longitudinal controller in AoA/3(Anti-windup A_w_z)
  A_w_z des/1 -> Longitudinal controller in AoA/1(A_w_z des)
  Sum/1 -> "Display4 "/1, "Sigmoid "/1(In), Physical limitation/1(v comm)  "v"
  All measures/1 -> Complete crossed On-line (adaptive) multi-layer NN: AoA/2(All_meas), Longitudinal controller in AoA/5(All meas), Physical limitation/2(all meas), Body Rates Controller/4(All_meas), Lat_dir Dyn Inversion: beta_dot->r_c/2(All_meas), Bus Selector3/1, Long Dyn Inversion: alpha_dot ->q/2(All_meas)
  Body Rates Controller/4(Angular acc des (rad/s^2)) -> Display3/1, Sum/2  "v_p+v_dot_ff"
  Bus Creator/1 -> Complete crossed On-line (adaptive) multi-layer NN: AoA/3(NN variables)
  Memory/1 -> Complete crossed On-line (adaptive) multi-layer NN: AoA/1(v_ad^ prev)
  Body Rates Controller/2(p_chanel vars) -> Bus Creator/2  "p_chanel_vars"
  Body Rates Controller/1(q_chanel vars) -> Bus Creator1/2  "q_chanel_vars"
  Longitudinal controller in AoA/1(alpha_chanel vars) -> Bus Creator1/1  "alpha_chanel vars"
  Bus Creator1/1 -> Bus Creator/1  "Long chanel"
  Ref Model and P Controller/2 -> Bus Creator2/1  "beta_sf_dot"
  Ref Model and P Controller/3 -> Sum1/1, Bus Creator2/2  "beta_sf"
  Sum1/1 -> Bus Creator2/3  "beta_err"
  Ref Model and P Controller/4 -> Sum1/2
  Ref Model and P Controller/5 -> Bus Creator2/4  "K_b_beta"
  Body Rates Controller/3(r_chanel vars) -> Bus Creator3/1  "r_chanel vars"
  Bus Creator2/1 -> Bus Creator3/2  "beta_chanel vars"
  Bus Creator3/1 -> Bus Creator/3  "beta_r_chanel"
  Anti-windup beta/1 -> Terminator1/1
  "Sigmoid "/1(Out) -> Memory/1
  Complete crossed On-line (adaptive) multi-layer NN: AoA/1(v_ad^) -> Scope1/1, Display2/1, Sum/1  "v_ad^"
  Ref Model and P Controller/1 -> Display5/1, Lat_dir Dyn Inversion: beta_dot->r_c/1(beta_dot_c)
  Physical limitation/1(v limted) -> Angular acc des/1
  Anti-windup signals/1 -> Complete crossed On-line (adaptive) multi-layer NN: AoA/4(AWU)
  Active/1 -> Complete crossed On-line (adaptive) multi-layer NN: AoA/Enable

== system F16ASYM_Controlled_AoA/Primary Controller/P  + Crossed NN + AWU+Lim + hand-over/Transitions Smotother  ==
  From AoA : Inport
  Indicator : Inport  Port=2
  From  ACC : Inport  Port=3
  "ACC -> AoA" : Saturate  UpperLimit=1  LowerLimit=0
  Abs : Abs
  Abs1 : Abs
  Add : Sum  Inputs=+-  OutDataTypeStr=double
  Add{1,4,6..7} (4 alike) : Sum  Inputs=+-
  Add2 : Sum  Inputs=-+
  Add3 : Sum  Inputs=-+
  "AoA -> ACC" : Saturate  UpperLimit=0  LowerLimit=-1
  Divide : Product  Inputs=**
  Divide1 : Product  Inputs=**
  Gain1 : Gain  Gain=-1/5
  Gain2 : Gain  Gain=-1/5
  Integrator Limited1 : Integrator  ExternalReset=level  InitialConditionSource=external  LimitOutput=on  UpperSaturationLimit=100  LowerSaturationLimit=-100
  Integrator Limited2 : Integrator  ExternalReset=level  InitialConditionSource=external  LimitOutput=on  UpperSaturationLimit=100  LowerSaturationLimit=-100
  Logical Operator : Logic  Operator=NOT  IconShape=distinctive  AllPortsSameDT=off  OutDataTypeStr=boolean
  Logical Operator1 : Logic  Operator=NOT  IconShape=distinctive  AllPortsSameDT=off  OutDataTypeStr=boolean
  Logical Operator2 : Logic  Operator=NOT  IconShape=distinctive  AllPortsSameDT=off  OutDataTypeStr=boolean
  Sample and Hold{1..4} (4 alike) : dspsigops/Sample and Hold  trig=Either edge  initCond=0  latchinput=off
  Scope{1..4} (4 alike) : Scope
      Scope1 settings: SaveName=ScopeData35
      Scope2 settings: SaveName=ScopeData34
      Scope3 settings: SaveName=ScopeData36
      Scope4 settings: YMin=-0.08  YMax=0.02  SaveName=ScopeData37
  Switch : Switch  Threshold=0.5  InputSameDT=on
  Timer signal : Subsystem  mask{time_delay=5}
      mask prompts: time_delay "Time to delay (s)"
  Unit Delay : UnitDelay  SampleTime=-1
  Ang accels comm : Outport
  wires:
  Indicator/1 -> Switch/2, Unit Delay/1, Add/1
  Unit Delay/1 -> Add/2
  Abs1/1 -> Timer signal/1(Triger)
  Timer signal/1(Logic output) -> Logical Operator/1
  From  ACC/1 -> Add3/2, Add2/2, Add4/1, Sample and Hold4/1, Add1/2
  Add/1 -> "AoA -> ACC"/1, "ACC -> AoA"/1, Abs1/1
  "AoA -> ACC"/1 -> Abs/1
  Add1/1 -> Sample and Hold3/1
  From AoA/1 -> Sample and Hold2/1, Add2/1, Add7/1, Add6/1, Add1/1
  Abs/1 -> Sample and Hold1/Trigger, Sample and Hold2/Trigger
  Add2/1 -> Sample and Hold1/1
  Sample and Hold1/1 -> Integrator Limited1/3
  Add3/1 -> Gain1/1
  Sample and Hold2/1 -> Add3/1
  Integrator Limited1/1 -> Divide/2
  Add4/1 -> Switch/3
  Logical Operator/1 -> Integrator Limited2/2, Logical Operator2/1, Integrator Limited1/2, Logical Operator1/1, Scope2/1
  Switch/1 -> Scope1/1, Ang accels comm/1
  Add6/1 -> Switch/1
  Integrator Limited2/1 -> Divide1/2
  "ACC -> AoA"/1 -> Sample and Hold3/Trigger, Sample and Hold4/Trigger
  Sample and Hold4/1 -> Add7/2
  Sample and Hold3/1 -> Gain2/1, Integrator Limited2/3
  Gain1/1 -> Integrator Limited1/1
  Gain2/1 -> Integrator Limited2/1
  Logical Operator1/1 -> Divide/1
  Divide/1 -> Add4/2, Scope4/1
  Divide1/1 -> Scope3/1, Add6/2
  Logical Operator2/1 -> Divide1/1

== system F16ASYM_Controlled_AoA/Primary Controller/P  + Crossed NN + AWU+Lim + hand-over/Transitions Smotother 1 ==
  From AoA : Inport
  Indicator : Inport  Port=2
  From  ACC : Inport  Port=3
  "ACC -> AoA" : Saturate  UpperLimit=1  LowerLimit=0
  Abs : Abs
  Add : Sum  Inputs=+-  OutDataTypeStr=double
  Add1 : Sum  Inputs=+-
  Add2 : Sum  Inputs=-+
  Add3 : Sum  Inputs=+-
  Add5 : Sum  Inputs=+-
  "AoA -> ACC" : Saturate  UpperLimit=0  LowerLimit=-1
  Gain : Gain  Gain=-1/5
  Gain1 : Gain  Gain=-1/5
  Integrator Limited : Integrator  ExternalReset=rising  InitialConditionSource=external  LimitOutput=on  UpperSaturationLimit=10000  LowerSaturationLimit=0
  Integrator Limited1 : Integrator  ExternalReset=rising  InitialConditionSource=external  LimitOutput=on  UpperSaturationLimit=100  LowerSaturationLimit=0
  Sample and Hold1 : dspsigops/Sample and Hold  trig=Rising edge  initCond=0  latchinput=off
  Sample and Hold2 : dspsigops/Sample and Hold  trig=Rising edge  initCond=0  latchinput=off
  Scope4 : Scope
      settings: YMin=-4  YMax=1.5  SaveName=ScopeData38
  Switch : Switch  Threshold=0.5  InputSameDT=on
  Unit Delay : UnitDelay  SampleTime=-1
  Out1 : Outport
  wires:
  Switch/1 -> Out1/1
  Gain1/1 -> Integrator Limited1/1
  Gain/1 -> Integrator Limited/1
  Add5/1 -> Switch/3
  Sample and Hold1/1 -> Integrator Limited1/3, Gain1/1
  Abs/1 -> Integrator Limited1/2, Sample and Hold1/Trigger
  Integrator Limited1/1 -> Add5/2
  Add2/1 -> Sample and Hold1/1
  Add3/1 -> Switch/1
  Sample and Hold2/1 -> Integrator Limited/3, Gain/1
  "ACC -> AoA"/1 -> Integrator Limited/2, Sample and Hold2/Trigger
  Integrator Limited/1 -> Add3/2
  Add1/1 -> Sample and Hold2/1
  "AoA -> ACC"/1 -> Abs/1
  Add/1 -> "AoA -> ACC"/1, "ACC -> AoA"/1
  From  ACC/1 -> Add1/2, Add5/1, Add2/2
  From AoA/1 -> Add2/1, Add1/1, Add3/1, Scope4/1
  Unit Delay/1 -> Add/2
  Indicator/1 -> Add/1, Unit Delay/1, Switch/2

== system F16ASYM_Controlled_AoA/Primary Controller/P controller/Body Rates Controller ==
  p_ref : Inport
  q_ref : Inport  Port=2
  r_ref : Inport  Port=3
  All_meas : Inport  Port=4
  Bus Creator : BusCreator
  Bus Creator1 : BusCreator
  Bus Creator2 : BusCreator
  Bus Selector : BusSelector  OutputSignals=signal1.omega_b meas (rad/s)
  Display1 : Display
  Mux : Mux  Inputs=3
  Ref Model and P Controller p : Adaptive_FaultTolerantControl/Ref Model and P Controller  tau=0.1  y_i=trim_state(10)  K_f=1  K_b=7
  Ref Model and P Controller q : Adaptive_FaultTolerantControl/Ref Model and P Controller  tau=0.06  y_i=trim_state(11)  K_f=1  K_b=1
  Ref Model and P Controller r : Adaptive_FaultTolerantControl/Ref Model and P Controller  tau=0.2  y_i=trim_state(12)  K_f=1  K_b=3
  Selector : Selector  InputPortWidth=3  IndexOptions=Index vector (dialog)  Indices=1  OutputSizes=1
  Selector1 : Selector  InputPortWidth=3  IndexOptions=Index vector (dialog)  Indices=2  OutputSizes=1
  Selector2 : Selector  InputPortWidth=3  IndexOptions=Index vector (dialog)  Indices=3  OutputSizes=1
  Sum : Sum  Inputs=+-|
  Sum1 : Sum  Inputs=+-|
  Sum2 : Sum  Inputs=+-|
  Terminator1 : Terminator
  Terminator2 : Terminator
  Terminator3 : Terminator
  Angular acc des (rad/s^2) : Outport
  wires:
  Ref Model and P Controller r/5 -> Bus Creator2/4  "K_b_r"
  Ref Model and P Controller r/4 -> Sum2/2
  Sum2/1 -> Bus Creator2/3  "p_err"
  Ref Model and P Controller r/3 -> Bus Creator2/2, Sum2/1  "p_sf"
  Ref Model and P Controller r/2 -> Bus Creator2/1  "p_sf_dot"
  Ref Model and P Controller q/5 -> Bus Creator1/4  "K_b_q"
  Ref Model and P Controller q/4 -> Sum1/2
  Sum1/1 -> Bus Creator1/3  "p_err"
  Ref Model and P Controller q/3 -> Bus Creator1/2, Sum1/1  "p_sf"
  Ref Model and P Controller q/2 -> Bus Creator1/1  "p_sf_dot"
  Ref Model and P Controller p/5 -> Bus Creator/4  "K_b_p"
  Ref Model and P Controller p/4 -> Sum/2
  Selector2/1 -> Ref Model and P Controller r/2
  Bus Creator2/1 -> Terminator3/1
  Bus Creator1/1 -> Terminator1/1
  Bus Creator/1 -> Terminator2/1
  Sum/1 -> Bus Creator/3, Display1/1  "p_err"
  Ref Model and P Controller p/3 -> Bus Creator/2, Sum/1  "p_sf"
  Ref Model and P Controller p/2 -> Bus Creator/1  "p_sf_dot"
  Ref Model and P Controller r/1 -> Mux/3
  Ref Model and P Controller q/1 -> Mux/2
  r_ref/1 -> Ref Model and P Controller r/1
  Selector1/1 -> Ref Model and P Controller q/2
  q_ref/1 -> Ref Model and P Controller q/1
  Mux/1 -> Angular acc des (rad/s^2)/1
  Ref Model and P Controller p/1 -> Mux/1
  Selector/1 -> Ref Model and P Controller p/2
  p_ref/1 -> Ref Model and P Controller p/1
  Bus Selector/1 -> Selector2/1, Selector1/1, Selector/1  "<omega_b meas (rad/s)>"
  All_meas/1 -> Bus Selector/1

== system F16ASYM_Controlled_AoA/Primary Controller/P controller/Lat_dir Dyn Inversion: beta_dot->r_c ==
  beta_dot_c : Inport
  All_meas : Inport  Port=2
  A_w_y : Selector  InputPortWidth=3  IndexOptions=Index vector (dialog)  Indices=2  OutputSizes=1
  Bus Selector : BusSelector  OutputSignals=signal1.AoA meas (rad),signal1.omega_b meas (rad/s),signal1.V_TAS (m/s),signal2.A_w_CG
  Divide1 : Product  Inputs=**
  Divide3 : Product  Inputs=**
  Divide4 : Product  Inputs=/*
  Divide5 : Product  Inputs=*/
  Selector : Selector  InputPortWidth=3  IndexOptions=Index vector (dialog)  Indices=1  OutputSizes=1
  Trigonometric Function : Trigonometry  Operator=cos
  Trigonometric Function3 : Trigonometry  Operator=tan
  "q_c " : Sum  Inputs=-++
  r_c : Outport
  wires:
  Selector/1 -> Divide1/2
  Trigonometric Function3/1 -> Divide1/1
  beta_dot_c/1 -> Divide5/1
  Divide5/1 -> "q_c "/1
  Trigonometric Function/1 -> Divide5/2, Divide3/1
  Bus Selector/3 -> Divide3/2  "<V_TAS (m/s)>"
  Divide4/1 -> "q_c "/3
  Bus Selector/4 -> A_w_y/1  "<A_w_CG>"
  All_meas/1 -> Bus Selector/1
  A_w_y/1 -> Divide4/2
  Divide3/1 -> Divide4/1
  Divide1/1 -> "q_c "/2
  Bus Selector/2 -> Selector/1  "<omega_b meas (rad/s)>"
  Bus Selector/1 -> Trigonometric Function3/1, Trigonometric Function/1  "<AoA meas (rad)>"
  "q_c "/1 -> r_c/1

== system F16ASYM_Controlled_AoA/Primary Controller/P controller/Long Dyn Inversion: alpha_dot ->q ==
  alpha_dot_c : Inport
  All_meas : Inport  Port=2
  Completed : Subsystem
  Manual Switch : ManualSwitch
  Simplified : Subsystem
  q_c : Outport
  wires:
  Manual Switch/1 -> q_c/1
  Simplified/1(q_c) -> Manual Switch/2
  Completed/1(q_c) -> Manual Switch/1
  All_meas/1 -> Completed/2(All_meas), Simplified/2(All_meas)
  alpha_dot_c/1 -> Completed/1(alpha_dot_c), Simplified/1(alpha_dot_c)

== system F16ASYM_Controlled_AoA/Primary Controller/P controller/Longitudinal Controller: AoA or A_w_z ==
  A_w_z des : Inport
  AoA des (rad) : Inport  Port=2
  Anti-windup A_w_z : Inport  Port=3
  Anti-windup AoA : Inport  Port=4
  All meas : Inport  Port=5
  Longitudinal controller in A_w_z : Subsystem  VariantObject=Controller of A_w_z
  Longitudinal controller in AoA : Subsystem  VariantObject=Controller of AoA
  A_chanel vars : Outport
  alpha_chanel vars : Outport  Port=2
  alpha_dot_c : Outport  Port=3

== system F16ASYM_Controlled_AoA/Primary Controller/P controller + adaptive Crossed NN/Body Rates Controller ==
  p_ref : Inport
  q_ref : Inport  Port=2
  r_ref : Inport  Port=3
  All_meas : Inport  Port=4
  Bus Creator : BusCreator
  Bus Creator1 : BusCreator
  Bus Creator2 : BusCreator
  Bus Selector : BusSelector  OutputSignals=signal1.omega_b meas (rad/s)
  Display1 : Display
  Mux : Mux  Inputs=3
  Ref Model and P Controller p : Adaptive_FaultTolerantControl/Ref Model and P Controller  tau=0.1  y_i=trim_state(10)  K_f=1  K_b=7
  Ref Model and P Controller q : Adaptive_FaultTolerantControl/Ref Model and P Controller  tau=0.25  y_i=trim_state(11)  K_f=1  K_b=7
  Ref Model and P Controller r : Adaptive_FaultTolerantControl/Ref Model and P Controller  tau=0.2  y_i=trim_state(12)  K_f=1  K_b=4
  Selector : Selector  InputPortWidth=3  IndexOptions=Index vector (dialog)  Indices=1  OutputSizes=1
  Selector1 : Selector  InputPortWidth=3  IndexOptions=Index vector (dialog)  Indices=2  OutputSizes=1
  Selector2 : Selector  InputPortWidth=3  IndexOptions=Index vector (dialog)  Indices=3  OutputSizes=1
  Sum : Sum  Inputs=+-|
  Sum1 : Sum  Inputs=+-|
  Sum2 : Sum  Inputs=+-|
  q_chanel vars : Outport
  p_chanel vars : Outport  Port=2
  r_chanel vars : Outport  Port=3
  Angular acc des (rad/s^2) : Outport  Port=4
  wires:
  Ref Model and P Controller r/5 -> Bus Creator2/4  "K_b_r"
  Ref Model and P Controller r/4 -> Sum2/2
  Sum2/1 -> Bus Creator2/3  "r_err"
  Ref Model and P Controller r/3 -> Bus Creator2/2, Sum2/1  "r_sf"
  Ref Model and P Controller r/2 -> Bus Creator2/1  "r_sf_dot"
  Ref Model and P Controller q/5 -> Bus Creator1/4  "K_b_q"
  Ref Model and P Controller q/4 -> Sum1/2
  Sum1/1 -> Bus Creator1/3  "q_err"
  Ref Model and P Controller q/3 -> Bus Creator1/2, Sum1/1  "q_sf"
  Ref Model and P Controller q/2 -> Bus Creator1/1  "q_sf_dot"
  Ref Model and P Controller p/5 -> Bus Creator/4  "K_b_p"
  Ref Model and P Controller p/4 -> Sum/2
  Selector2/1 -> Ref Model and P Controller r/2
  Bus Creator2/1 -> r_chanel vars/1
  Bus Creator1/1 -> q_chanel vars/1
  Bus Creator/1 -> p_chanel vars/1
  Sum/1 -> Bus Creator/3, Display1/1  "p_err"
  Ref Model and P Controller p/3 -> Bus Creator/2, Sum/1  "p_sf"
  Ref Model and P Controller p/2 -> Bus Creator/1  "p_sf_dot"
  Ref Model and P Controller r/1 -> Mux/3
  Ref Model and P Controller q/1 -> Mux/2
  r_ref/1 -> Ref Model and P Controller r/1
  Selector1/1 -> Ref Model and P Controller q/2
  q_ref/1 -> Ref Model and P Controller q/1
  Mux/1 -> Angular acc des (rad/s^2)/1
  Ref Model and P Controller p/1 -> Mux/1
  Selector/1 -> Ref Model and P Controller p/2
  p_ref/1 -> Ref Model and P Controller p/1
  Bus Selector/1 -> Selector2/1, Selector1/1, Selector/1  "<omega_b meas (rad/s)>"
  All_meas/1 -> Bus Selector/1

== system F16ASYM_Controlled_AoA/Primary Controller/P controller + adaptive Crossed NN/Complete crossed On-line (adaptive) multi-layer NN ==
  v_ad^ prev : Inport
  All_meas : Inport  Port=2
  NN variables : Inport  Port=3
  Complete crossed On-line (adaptive) multi-layer NN: A_w_z : Subsystem  VariantObject=NN on A_w_z
  Complete crossed On-line (adaptive) multi-layer NN: AoA : Subsystem  VariantObject=NN on AoA
  v_ad^ : Outport
